simulink model "untitled1"  (R2014b)
settings: Solver=ode45  StartTime=0.0  StopTime=10.0  RelTol=1e-3
settings Model: Creator=rajab  LastModifiedBy=rajab

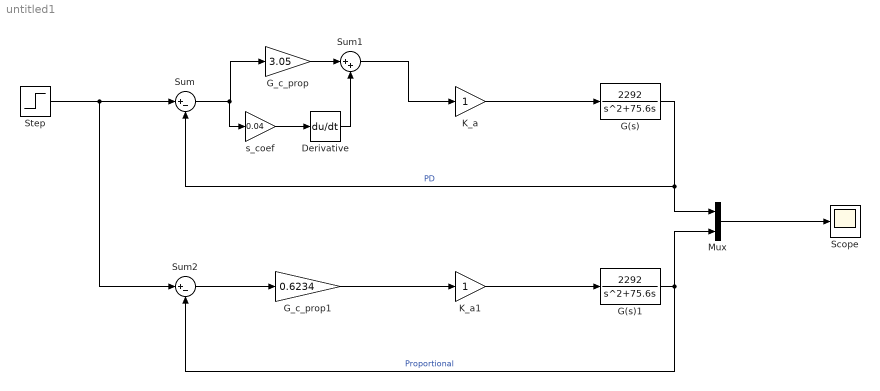
== system untitled1 ==
  Derivative : Derivative
  G(s) : TransferFcn  Numerator=[2292]  Denominator=[1 75.6 0]
  G(s)1 : TransferFcn  Numerator=[2292]  Denominator=[1 75.6 0]
  G_c_prop : Gain  Gain=3.05
  G_c_prop1 : Gain  Gain=0.6234
  K_a : Gain
  K_a1 : Gain
  Mux : Mux  Inputs=2
  Scope : Scope
      settings: ShowLegends=on
  Step : Step  SampleTime=0
  Sum : Sum  Inputs=|+-
  Sum1 : Sum  Inputs=|++
  Sum2 : Sum  Inputs=|+-
  s_coef : Gain  Gain=0.04
  wires:
  K_a/1 -> G(s)/1
  G(s)/1 -> Mux/1, Sum/2  "PD"
  Sum/1 -> s_coef/1, G_c_prop/1
  G_c_prop/1 -> Sum1/1
  Derivative/1 -> Sum1/2
  Sum1/1 -> K_a/1
  s_coef/1 -> Derivative/1
  K_a1/1 -> G(s)1/1
  G(s)1/1 -> Sum2/2, Mux/2  "Proportional"
  Sum2/1 -> G_c_prop1/1
  Step/1 -> Sum2/1, Sum/1
  G_c_prop1/1 -> K_a1/1
  Mux/1 -> Scope/1
